simulink model "Landing_Station_Following_Drone"  (R2024b)
settings: Solver=ode3  StartTime=0  StopTime=TFinal  FixedStep=Ts  RelTol=1e-3  EnableMultiTasking=on
model workspace (MAT data in the model file):
  CIRCLE_PTS = [19 19 19]
  ZEROS = [0 0 0 0 0 0 0 0 0 0 0 0 ... (1444 elements, 38x38)]
undefined symbols (not defined in the file): codertarget, Controller, DiscIntNeverNeededParam, Discrete, Estimator, g, gray, init, orient_ref, pos_ref, Sensors, Time, Ts, var_acc_angle_N, var_bias_gyr_N, var_gyro_p_N, Vehicle
libraries: simulink x42, slpidlib x4, ctrlSharedLib x4, matrix_library x4, sharedtransform x3, parrotlib x1
(part 3 of 3)

== matlab function Landing_Station_Following_Drone/Image Processing System/MATLAB Function3 ==
  data: flag input; R input; BW output; G input; B input
function BW  = createMask(flag,R,G,B)
%createMask  Threshold RGB image using auto-generated code from colorThresholder app.
%  [BW,MASKEDRGBIMAGE] = createMask(RGB) thresholds image RGB using
%  auto-generated code from the colorThresholder app. The colorspace and
%  range for each channel of the colorspace were set within the app. The
%  segmentation mask is returned in BW, and a composite of the mask and
%  original RGB images is returned in maskedRGBImage.

% Auto-generated by colorThresholder app on 03-Feb-2024
%------------------------------------------------------

I = cat(3,R,G,B)
HSV = rgb2hsv(I)
[H,S,V] = imsplit(HSV)

% Convert RGB image to chosen color space

if flag == 1
% Define thresholds for channel 1 based on histogram settings
channel1Min = 125.000;
channel1Max = 173.000;

% Define thresholds for channel 2 based on histogram settings
channel2Min = 180.000;
channel2Max = 255.000;

% Define thresholds for channel 3 based on histogram settings
channel3Min = 98.000;
channel3Max = 155.000;




% Create mask based on chosen histogram thresholds
sliderBW = (R >= channel1Min ) & (R <= channel1Max) & ...
    (G >= channel2Min ) & (G <= channel2Max) & ...
    (B >= channel3Min ) & (B <= channel3Max);
BW = sliderBW;


elseif flag ==2
% Define thresholds for channel 1 based on histogram settings
channel1Min = 0.894;
channel1Max = 0.002;

% Define thresholds for channel 2 based on histogram settings
channel2Min = 0.180;
channel2Max = 0.628;

% Define thresholds for channel 3 based on histogram settings
channel3Min = 0.463;
channel3Max = 1.000;



sliderBW = ( H >= channel1Min) | (H <= channel1Max)  & ...
    (S >= channel2Min ) & (S <= channel2Max) & ...
    (V >= channel3Min ) & (V <= channel3Max);
BW = sliderBW;
elseif flag == 3
% Define thresholds for channel 1 based on histogram settings
channel1Min = 0.929;
channel1Max = 0.986;

% Define thresholds for channel 2 based on histogram settings
channel2Min = 0.285;
channel2Max = 0.567;

% Define thresholds for channel 3 based on histogram settings
channel3Min = 0.500;
channel3Max = 1.000;





% Create mask based on chosen histogram thresholds
sliderBW = (H >= channel1Min ) | (H <= channel1Max) & ...
    (S >= channel2Min ) & (S <= channel2Max) & ...
    (V >= channel3Min ) & (V <= channel3Max);
BW = sliderBW;
elseif flag == 4
% Define thresholds for channel 1 based on histogram settings
channel1Min = 0.118;
channel1Max = 0.183;

% Define thresholds for channel 2 based on histogram settings
channel2Min = 0.122;
channel2Max = 1.000;

% Define thresholds for channel 3 based on histogram settings
channel3Min = 0.852;
channel3Max = 1.000;





% Create mask based on chosen histogram thresholds
sliderBW = (H >= channel1Min ) & (H <= channel1Max) & ...
    (S >= channel2Min ) & (S <= channel2Max) & ...
    (V >= channel3Min ) & (V <= channel3Max);
BW = sliderBW;
else
       % Define thresholds for channel 1 based on histogram settings
channel1Min = 236.000;
channel1Max = 255.000;

% Define thresholds for channel 2 based on histogram settings
channel2Min = 0.000;
channel2Max = 255.000;

% Define thresholds for channel 3 based on histogram settings
channel3Min = 0.000;
channel3Max = 255.000;


% Create mask based on chosen histogram thresholds
sliderBW = (R >= channel1Min ) & (R <= channel1Max) & ...
    (G >= channel2Min ) & (G <= channel2Max) & ...
    (B >= channel3Min ) & (B <= channel3Max);
BW = sliderBW;
    BW = sliderBW
end

end
